simulink model "testStarTracker"  (R2021a)
settings: Solver=VariableStepAuto  StartTime=0.0  StopTime=10.0  RelTol=1e-3
settings Model: Creator=jmher  LastModifiedBy=jmher

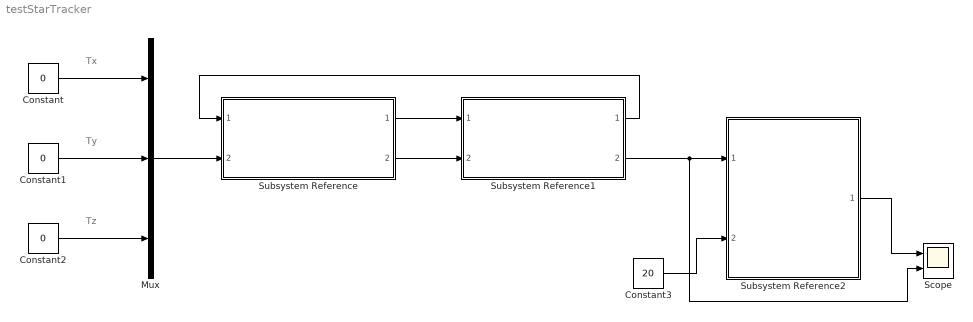
== system testStarTracker ==
  note: Tx
  note: Ty
  note: Tz
  Constant : Constant  Value=0
  Constant1 : Constant  Value=0
  Constant2 : Constant  Value=0
  Constant3 : Constant  Value=20
  Mux : Mux  Inputs=3
  Scope : Scope  NumInputPorts=2
  Subsystem Reference : Subsystem  ReferencedSubsystem=Dynamics
  Subsystem Reference1 : Subsystem  ReferencedSubsystem=Kinematics
  Subsystem Reference2 : Subsystem  ReferencedSubsystem=StarTracker
  wires:
  Constant2/1 -> Mux/3
  Mux/1 -> Subsystem Reference/2
  Subsystem Reference/2 -> Subsystem Reference1/2
  Constant1/1 -> Mux/2
  Subsystem Reference1/2 -> Scope/2, Subsystem Reference2/1
  Subsystem Reference/1 -> Subsystem Reference1/1
  Subsystem Reference1/1 -> Subsystem Reference/1
  Constant/1 -> Mux/1
  Constant3/1 -> Subsystem Reference2/2
  Subsystem Reference2/1 -> Scope/1
